simulink model "blabla"  (R2021a)
settings: Solver=VariableStepAuto  StartTime=0.0  StopTime=1  RelTol=1e-3
libraries: spsSeriesRLCBranchLib x3, spsVoltageMeasurementLib x2, spsDCVoltageSourceLib x1, spsDiodeLib x1, spsIGBTDiodeLib x1, spsPWMGeneratorDCDCLib x1, spspowerguiLib x1
settings Model: Creator=Asus  LastModifiedBy=User

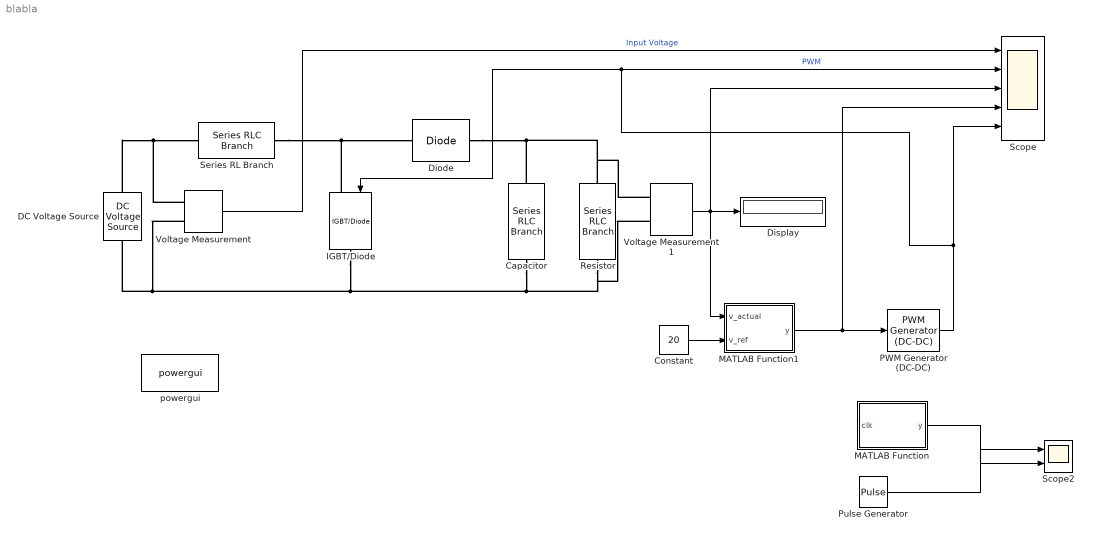
== system blabla ==
  Capacitor : spsSeriesRLCBranchLib/Series RLC Branch  LConnTagsString=__new0  RConnTagsString=__new0  BranchType=C  Resistance=1  Inductance=1e-3  SetiL0=off  InitialCurrent=0  Capacitance=1000e-6  Setx0=off  InitialVoltage=0  Measurements=None
  Constant : Constant  Value=20
  DC Voltage Source : spsDCVoltageSourceLib/DC Voltage Source  Amplitude=10  Measurements=None
  Diode : spsDiodeLib/Diode  Ron=0.001  Lon=0  Vf=0.8  IC=0  UseSnubber=0  Rs=500  Cs=250e-9  Measurements=off
  Display : Display
  IGBT/Diode : spsIGBTDiodeLib/IGBT//Diode  Ron=1e-3  Rs=1e5  Cs=inf  Measurements=off
  MATLAB Function : MATLAB Function  TreatAsAtomicUnit=on
  MATLAB Function1 : MATLAB Function  TreatAsAtomicUnit=on
  PWM Generator (DC-DC) : spsPWMGeneratorDCDCLib/PWM Generator (DC-DC)  Fsw=5000  Ts=0
  Pulse Generator : DiscretePulseGenerator  PulseType=Time based  Period=.0002  PulseWidth=50
  Resistor : spsSeriesRLCBranchLib/Series RLC Branch  LConnTagsString=__new0  RConnTagsString=__new0  BranchType=R  Resistance=20  Inductance=1e-3  SetiL0=off  InitialCurrent=0  Capacitance=1e-6  Setx0=off  InitialVoltage=0  Measurements=None
  Scope : Scope  NumInputPorts=5
  Scope2 : Scope  NumInputPorts=2
  Series RL Branch : spsSeriesRLCBranchLib/Series RLC Branch  LConnTagsString=__new0  RConnTagsString=__new0  BranchType=RL  Resistance=.1  Inductance=10e-6  SetiL0=off  InitialCurrent=0  Capacitance=1e-6  Setx0=off  InitialVoltage=0  Measurements=None
  Voltage Measurement : spsVoltageMeasurementLib/Voltage Measurement  PhasorSimulation=off  OutputType=Complex  PSBequivalent=0
  Voltage Measurement1 : spsVoltageMeasurementLib/Voltage Measurement  PhasorSimulation=off  OutputType=Complex  PSBequivalent=0
  powergui : spspowerguiLib/powergui  Priority=1  SimulationMode=Discrete  SampleTime=50e-6  frequency=60  Iterations=50  frequencyindice=0  Pbase=100e6  ErrMax=1e-4  UnitsV=kV  UnitsW=MW  buscounter=0  FunctionMessages=off  echomessages=off  EnableUseOfTLC=off  CurrentSourceSwitches=off  DisableSnubberDevices=off  DisableRonSwitches=off  DisableVfSwitches=off  DisplayEquations=off  AutomaticDiscreteSolvers=off  SolverType=Tustin/Backward Euler (TBE)  Interpol=off  ExternalGateDelay=off  methode=off  Ts=100  x0status=blocks  SPID=on  SwTol=0  HookPort=off  NonlinearTolerance=1e-4  nMaxIteration=100  ContinueOnMaxIteration=off  RestoreLinks=warning  ResistiveCurrentMeasurement=off  Frange=[0:2:500]  Ylog=off  Xlog=on  ShowGrid=off  save=off  variable=ZData  structure=0  ZoomFFT=off  StartTime=0.0  cycles=1  DisplayStyle=1  fundamental=60  FreqAxis=off  MaxFrequency=1000  frequencyindicesteady=1  RmsSteady=1  display=off
  wires:
  Voltage Measurement/1 -> Scope/1  "Input Voltage"
  Constant/1 -> MATLAB Function1/2(v_ref)
  Voltage Measurement1/1 -> Scope/3, MATLAB Function1/1(v_actual), Display/1
  Pulse Generator/1 -> Scope2/1
  PWM Generator (DC-DC)/1 -> Scope/5, IGBT/Diode/1, Scope/2  "PWM"
  MATLAB Function1/1(y) -> PWM Generator (DC-DC)/1, Scope/4
  MATLAB Function/1(y) -> Scope2/2
  connections:
  DC Voltage Source/RConn1 -- Voltage Measurement/LConn1 -- Series RL Branch/LConn1
  Series RL Branch/RConn1 -- IGBT/Diode/LConn1 -- Diode/LConn1
  Capacitor/RConn1 -- Voltage Measurement1/LConn2 -- Resistor/RConn1 -- IGBT/Diode/RConn1 -- Voltage Measurement/LConn2 -- DC Voltage Source/LConn1
  Diode/RConn1 -- Resistor/LConn1 -- Voltage Measurement1/LConn1 -- Capacitor/LConn1

== matlab function blabla/MATLAB Function ==
  data: clk input; y output
function y = fcn(clk)

if clk <.1
    d = .2
elseif clk >=.1 && clk <.2
    d= .4
elseif clk >=.2 && clk <.3
    d=.6
elseif clk >=.3 && clk <.4
    d = .75
else
    d=.8
end
y = d;
end

== matlab function blabla/MATLAB Function1 ==
  settings: updateMethod=DISCRETE
  data: v_actual input; y output; v_ref input
function y = fcn(v_actual,v_ref)
delta = 0.01
persistent D
if isempty(D), D = .1; end
if v_actual < v_ref
    D = D+delta;
    if D>=.75
        D = .75;
    end
elseif v_actual > v_ref
    D = D-delta;
    if D<0;
        D = 0;
    end
else
    D = D;
end
y=D;
end
